simulink model "F4VGTx_ADC1_2ch_DMA"  (R2015b)
settings: Solver=FixedStepDiscrete  StartTime=0.0  StopTime=10.0  FixedStep=0.5  RelTol=1e-3
libraries: ADC_Lib x1, STM32_Config_Lib x1, USART_Lib x1
settings Model: Creator=reynaudp  LastModifiedBy=reynaudp
settings DataIOCC: SaveFormat=Array
settings OptimizationCC: OptimizeModelRefInitCode=on  LifeSpan=1
settings DebuggingCC: UnderspecifiedInitializationDetection=Classic  MergeDetectMultiDrivingBlocksExec=none  SolverPrmCheckMsg=warning
settings HardwareCC: ProdBitPerPointer=32  ProdLargestAtomicInteger=Integer  ProdWordSize=32  ProdHWDeviceType=STMicroelectronics->STM32 32-bit Cortex-M  TargetBitPerPointer=64  TargetLongLongMode=on  TargetIntDivRoundTo=Zero  TargetEndianess=LittleEndian  TargetWordSize=64  TargetHWDeviceType=MATLAB Host  ProdEqTarget=off
settings RTWCC: SystemTargetFile=stm32.tlc  TemplateMakefile=stm32.tmf  Description=stm32 (Embedded Target)  GenerateReport=on  IncludeHyperlinkInReport=on  LaunchReport=on
settings CodeAppCC: IgnoreCustomStorageClasses=off  MaxIdLength=64  CustomSymbolStrType=$N$R$M  SimulinkBlockComments=off
settings STFCustomTargetCC: ParMdlRefBuildCompliant=on  ConcurrentExecutionCompliant=off  IncludeMdlTerminateFcn=off  GeneratePreprocessorConditionals=Use local settings  CombineOutputUpdateFcns=on  ERTCustomFileBanners=on  SupportContinuousTime=off  SupportNonInlinedSFcns=off  MATLABClassNameForMDSCustomization=Simulink.SoftwareTarget.ERTCustomization  CPPClassGenCompliant=off  GRTInterface=off  SystemTargetFile=stm32.tlc
settings ERTTargetCC: CompOptLevelCompliant=off  ConcurrentExecutionCompliant=off  IncludeMdlTerminateFcn=off  ERTFirstTimeCompliant=off  ModelStepFunctionPrototypeControlCompliant=off  CPPClassGenCompliant=off  UseToolchainInfoCompliant=off  ERTSrcFileBannerTemplate=sourceFileTemplate.cgt  ERTHdrFileBannerTemplate=sourceFileTemplate.cgt  ERTDataSrcFileTemplate=sourceFileTemplate.cgt  ERTDataHdrFileTemplate=sourceFileTemplate.cgt  ERTCustomFileTemplate=customRoutineProcess.tlc
settings ConfigComp: CovModelRefEnable=Off  CovSFcnEnable=off

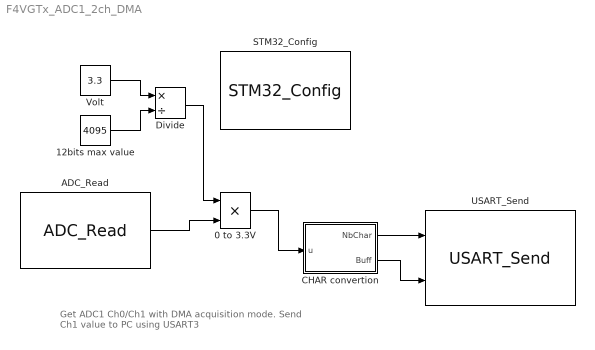
== system F4VGTx_ADC1_2ch_DMA ==
  note: Get ADC1 Ch0/Ch1 with DMA acquisition mode.
      | Send Ch1 value to PC using USART3
  0 to 3.3V : Product  RndMeth=Zero
  12bits max value : Constant  Value=4095
  ADC_Read : ADC_Lib/ADC_Read  ADC_Name=ADC1  ADC_Ch0=off  ADC_Ch1=on  ADC_Ch2=off  ADC_Ch3=off  ADC_Ch4=off  ADC_Ch5=off  ADC_Ch6=off  ADC_Ch7=off  ADC_Ch8=off  ADC_Ch9=off  ADC_Ch10=off  ADC_Ch11=off  ADC_Ch12=off  ADC_Ch13=off  ADC_Ch14=off  ADC_Ch15=off  ADC_Ch16=off  ADC_Ch17=off  ADC_Ch18=off  RgRk1=off  RgRk2=on  RgRk3=off  RgRk4=off  RgRk1_Ch=Ch0_r1  RgRk2_Ch=Ch1_r2  RgRk3_Ch=off  RgRk4_Ch=off  RgRk5=off  RgRk6=off  RgRk7=off  RgRk8=off  RgRk5_Ch=off  RgRk6_Ch=off  RgRk7_Ch=off  RgRk8_Ch=off  RgRk9=off  RgRk10=off  RgRk11=off  RgRk12=off  RgRk9_Ch=off  RgRk10_Ch=off  RgRk11_Ch=off  RgRk12_Ch=off  RgRk13=off  RgRk14=off  RgRk15=off  RgRk16=off  RgRk13_Ch=off  RgRk14_Ch=off  RgRk15_Ch=off  RgRk16_Ch=off  InjRk1=off  InjRk2=off  InjRk3=off  InjRk4=off  InjRk1_Ch=off  InjRk2_Ch=off  InjRk3_Ch=off  InjRk4_Ch=off  ADC_Trig=Not used  ADC_TrigEdge=Not used  DmaReq=on  ItReq=off  AWD_Mode=NOT_USED  AWD_Ch=0  AWD_HThres=0  AWD_LThres=0  AWD_En_Int=off  AWD2_HThres=0  AWD2_LThres=0  AWD2_En_Int=off  AWD3_HThres=0  AWD3_LThres=0  AWD3_En_Int=off  EOC_IT=off  JEOC_IT=off  AWD_IT=off  OVR_IT=off  ADC_RegNb=2  ADC_RegCh0=on  ADC_RegCh1=on  ADC_RegCh2=off  ADC_RegCh3=off  ADC_RegCh4=off  ADC_RegCh5=off  ADC_RegCh6=off  ADC_RegCh7=off  ADC_RegCh8=off  ADC_RegCh9=off  ADC_RegCh10=off  ADC_RegCh11=off  ADC_RegCh12=off  ADC_RegCh13=off  ADC_RegCh14=off  ADC_RegCh15=off  ADC_RegCh16=off  ADC_RegCh17=off  ADC_RegCh18=off  ADC_InjNb=0  ADC_InjCh0=off  ADC_InjCh1=off  ADC_InjCh2=off  ADC_InjCh3=off  ADC_InjCh4=off  ADC_InjCh5=off  ADC_InjCh6=off  ADC_InjCh7=off  ADC_InjCh8=off  ADC_InjCh9=off  ADC_InjCh10=off  ADC_InjCh11=off  ADC_InjCh12=off  ADC_InjCh13=off  ADC_InjCh14=off  ADC_InjCh15=off  ADC_InjCh16=off  ADC_InjCh17=off  ADC_InjCh18=off  ADC_RegRank0=1  ADC_RegRank1=2  ADC_RegRank2=0  ADC_RegRank3=0  ADC_RegRank4=0  ADC_RegRank5=0  ADC_RegRank6=0  ADC_RegRank7=0  ADC_RegRank8=0  ADC_RegRank9=0  ADC_RegRank10=0  ADC_RegRank11=0  ADC_RegRank12=0  ADC_RegRank13=0  ADC_RegRank14=0  ADC_RegRank15=0  ADC_RegRank16=0  ADC_RegRank17=0  ADC_RegRank18=0  ADC_InjRank0=0  ADC_InjRank1=0  ADC_InjRank2=0  ADC_InjRank3=0  ADC_InjRank4=0  ADC_InjRank5=0  ADC_InjRank6=0  ADC_InjRank7=0  ADC_InjRank8=0  ADC_InjRank9=0  ADC_InjRank10=0  ADC_InjRank11=0  ADC_InjRank12=0  ADC_InjRank13=0  ADC_InjRank14=0  ADC_InjRank15=0  ADC_InjRank16=0  ADC_InjRank17=0  ADC_InjRank18=0  NbADC=1  CurrentADC=ADC1
  CHAR convertion : MATLAB Function  TreatAsAtomicUnit=on
  Divide : Product  Inputs=*/
  STM32_Config : STM32_Config_Lib/STM32_Config  Priority=0  Project_Path=.\  Config_File=F4VGTx_ADC1_2ch_DMA.ioc  MCU_Name=STM32F407VGTx
  USART_Send : USART_Lib/USART_Send  USART_name=USART3  Buff_size=512  nbUsart=1  usartMode=Asynchronous  usartDma_Rx=off  usartDma_Tx=off  usartIt=on
  Volt : Constant  Value=3.3  OutDataTypeStr=single
  wires:
  Volt/1 -> Divide/1
  12bits max value/1 -> Divide/2
  Divide/1 -> 0 to 3.3V/1
  CHAR convertion/1(NbChar) -> USART_Send/1
  0 to 3.3V/1 -> CHAR convertion/1(u)
  CHAR convertion/2(Buff) -> USART_Send/2
  ADC_Read/1 -> 0 to 3.3V/2

== matlab function F4VGTx_ADC1_2ch_DMA/CHAR convertion ==
  data: u input; NbChar output uint16 size=1; Buff output uint32 size=1
function [NbChar, Buff] = convert(u)
if coder.target('Sfun')
% Executing in MATLAB, Buff is null
Buff = uint32(0);
NbChar = uint16(0);
else
% Executing in the generated code. 
buffer = zeros(1,15,'uint8');
strLen = int32(0);
strLen = coder.ceval('sprintf',coder.wref(buffer),['%2.2f',0],u);
%tmp = buffer(1:strLen);
tmp = uint8('Volt');
y = [buffer(1:4), tmp, 13, 10, 0];
%Buff = uint32(coder.ref(y));
Buff = coder.ceval('getBuffPtr',coder.ref(y));
NbChar = uint16(size(y,2));
end
end
%Buff = uint32(y);
%%Buff = [buffer(1:4), tmp, 13, 10, 0];
